simulink model "lab9"  (R2020b)
settings: Solver=VariableStepAuto  StartTime=0.0  StopTime=10.0  RelTol=1e-3
libraries: mpclib x1
settings Model: Creator=karth  LastModifiedBy=karth

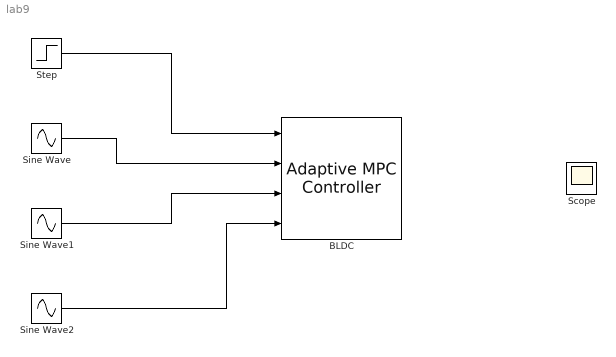
== system lab9 ==
  BLDC : mpclib/Adaptive MPC Controller  SCDEnableBlockLinearizationSpecification=on  enable_value=0  updateMPCinCallerWorkspace=on  md_inport=on  mv_inport=off  uref_inport=off  return_cost=off  return_mvseq=off  return_qpstatus=off  return_xseq=off  return_state=off  return_ovseq=off  state_inport=off  isltv_plant=off  umin_inport=off  umax_inport=off  ymin_inport=off  ymax_inport=off  cc_inport=off  ywt_inport=off  uwt_inport=off  duwt_inport=off  rhoeps_inport=off  pm_inport=off  MaximumP=10  HorizonChoice=FixedHorizon  BlockDataType=double  SampleTimeInherited=off  switch_inport=off
  Scope : Scope
  Sine Wave : Sin  SampleTime=0
  Sine Wave1 : Sin  SampleTime=0
  Sine Wave2 : Sin  SampleTime=0
  Step : Step  SampleTime=0
  wires:
  Step/1 -> BLDC/1
  Sine Wave/1 -> BLDC/2
  Sine Wave1/1 -> BLDC/3
  Sine Wave2/1 -> BLDC/4
